simulink model "aircraftPitch"  (R2019b)
settings: Solver=VariableStepAuto  StartTime=0.0  StopTime=10.0  RelTol=1e-3
settings Model: Creator=zhaoyuan_huo  LastModifiedBy=zhaoyuan_huo

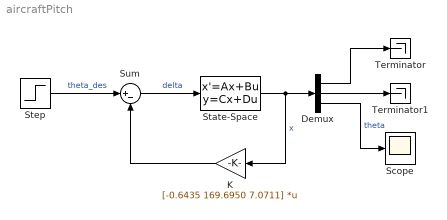
== system aircraftPitch ==
  Demux : Demux  Outputs=3
  K : Gain  Gain=[-0.6435 169.6950 7.0711]  Multiplication=Matrix(K*u)
  Scope : Scope
  State-Space : StateSpace  A=[-0.313 56.7 0; -0.0139 -0.426 0; 0 56.7 0]  B=[0.232; 0.0203; 0]  C=eye(3)  D=[0; 0; 0]  InitialCondition=0  ContinuousStateAttributes={'Angle_of_attack', 'Pitch_rate', 'Pitch_angle'}
  Step : Step  Time=0  After=0.2  SampleTime=0
  Sum : Sum  Inputs=|+-
  Terminator : Terminator
  Terminator1 : Terminator
  wires:
  Demux/3 -> Scope/1  "theta"
  Demux/1 -> Terminator/1
  Demux/2 -> Terminator1/1
  State-Space/1 -> K/1, Demux/1  "x"
  Step/1 -> Sum/1  "theta_des"
  Sum/1 -> State-Space/1  "delta"
  K/1 -> Sum/2
